simulink model "Copter_Plane_h2g_4_and_1"  (R2020a)
settings: Solver=ode1  StartTime=0.0  StopTime=100  FixedStep=dt  RelTol=1e-3
undefined symbols (not defined in the file or in its folder): center_WP, GRAVITY_MSS, gyro_x, gyro_y, gyro_z, HD, J, Kd, Ku, Ld, Ldx, Ldy, Lu, Lux, Luy, m_kg, Newton, pitch, pwm_max, pwm_min, Qd, QLd, QLdx, QLdy, QLu, QLux, QLuy, Qu, Raphson, roll, vel_desired, yaw
libraries: shared6dofsys x3, sharedutil x1, simulink x1, aerolibasang x1
(part 1 of 4)
settings Model: xpc_rtwmakecfg_data=_xpcnblib_  PauseTimes=2  Creator=a4327  LastModifiedBy=a4327
settings DataIOCC: ReturnWorkspaceOutputs=off
settings OptimizationCC: DefaultParameterBehavior=Inlined  UseDivisionForNetSlopeComputation=on  GainParamInheritBuiltInType=on  UseFloatMulNetSlope=on  InlineInvariantSignals=on  PassReuseOutputArgsAs=Individual arguments  ZeroExternalMemoryAtStartup=off  ZeroInternalMemoryAtStartup=off  NoFixptDivByZeroProtection=on  EfficientFloat2IntCast=on  LifeSpan=1  OptimizeBlockOrder=speed  DifferentSizesBufferReuse=on  EfficientTunableParamExpr=on
settings DebuggingCC: ParameterTunabilityLossMsg=error  ArithmeticOperatorsInVariantConditions=warning
settings HardwareCC: ProdBitPerPointer=32  ProdBitPerSizeT=32  ProdBitPerPtrDiffT=32  ProdLargestAtomicFloat=None  ProdWordSize=32  ProdLongLongMode=on  ProdHWDeviceType=Custom Processor->Custom Processor
settings SFSimCC: MATLABDynamicMemAlloc=off  CustomCodeUndefinedFunction=UseInterfaceOnly
settings RTWCC: SystemTargetFile=ert.tlc  TemplateMakefile=ert_default_tmf  GenerateReport=on  IncludeHyperlinkInReport=on  LaunchReport=on  GenerateTraceInfo=on  GenerateTraceReport=on  GenerateTraceReportSl=on  GenerateTraceReportSf=on  GenerateTraceReportEml=on  GenerateCodeMetricsReport=on
settings CodeAppCC: ForceParamTrailComments=on  IgnoreCustomStorageClasses=off  OperatorAnnotations=on  SimulinkDataObjDesc=on  SFDataObjDesc=on  CustomSymbolStrGlobalVar=rt$N$M  CustomSymbolStrType=$N$M  CustomSymbolStrFcn=$N$M$F  CustomSymbolStrMacro=$N$M  InsertBlockDesc=on
settings ERTTargetCC: TargetLangStandard=C99 (ISO)  GenerateSampleERTMain=on  IncludeMdlTerminateFcn=off  CombineSignalStateStructs=on  MultiInstanceERTCode=on  CodeInterfacePackaging=Reusable function  SupportComplex=off  SupportNonInlinedSFcns=on  InlinedParameterPlacement=NonHierarchical  RootIOFormat=Structure reference  ERTCustomFileTemplate=example_file_process.tlc  ERTFilePackagingFormat=CompactWithDataFile

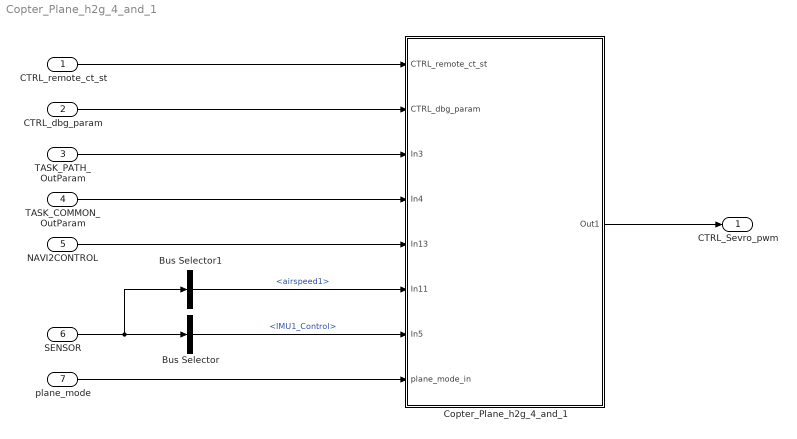
== system Copter_Plane_h2g_4_and_1 ==
  CTRL_remote_ct_st : Inport  OutDataTypeStr=Bus: BUS_CTRL_remote_ct_st  BusOutputAsStruct=on
  CTRL_dbg_param : Inport  Port=2  OutDataTypeStr=Bus: BUS_CTRL_dbg_param  BusOutputAsStruct=on
  TASK_PATH_OutParam : Inport  Port=3  OutDataTypeStr=Bus: BUS_TASK_PATH_OutParam  BusOutputAsStruct=on
  TASK_COMMON_OutParam : Inport  Port=4  OutDataTypeStr=Bus: BUS_TASK_COMMON_OutParam  BusOutputAsStruct=on
  NAVI2CONTROL : Inport  Port=5  OutDataTypeStr=Bus: BUS_TO_CONTROL  BusOutputAsStruct=on
  SENSOR : Inport  Port=6  OutDataTypeStr=Bus: BUS_SENSOR
  plane_mode : Inport  Port=7  OutDataTypeStr=Enum: ENUM_plane_mode
  Bus Selector : BusSelector  OutputSignals=IMU1_Control
  Bus Selector1 : BusSelector  OutputSignals=airspeed1
  Copter_Plane_h2g_4_and_1 : Subsystem
  CTRL_Sevro_pwm : Outport  OutDataTypeStr=Bus: BUS_CTRL_Sevro_pwm
  wires:
  CTRL_remote_ct_st/1 -> Copter_Plane_h2g_4_and_1/1(CTRL_remote_ct_st)
  Copter_Plane_h2g_4_and_1/1(Out1) -> CTRL_Sevro_pwm/1
  CTRL_dbg_param/1 -> Copter_Plane_h2g_4_and_1/2(CTRL_dbg_param)
  TASK_PATH_OutParam/1 -> Copter_Plane_h2g_4_and_1/3(In3)
  Bus Selector1/1 -> Copter_Plane_h2g_4_and_1/6(In11)  "<airspeed1>"
  SENSOR/1 -> Bus Selector1/1, Bus Selector/1
  TASK_COMMON_OutParam/1 -> Copter_Plane_h2g_4_and_1/4(In4)
  NAVI2CONTROL/1 -> Copter_Plane_h2g_4_and_1/5(In13)
  plane_mode/1 -> Copter_Plane_h2g_4_and_1/8(plane_mode_in)
  Bus Selector/1 -> Copter_Plane_h2g_4_and_1/7(In5)  "<IMU1_Control>"
